simulink model "tenzo1_05"  (Simulink 7.9)
settings: Solver=ode45  StartTime=0.0  StopTime=20  RelTol=1e-3
values from neighbouring files (symbols this model uses):
  A = [0 0 0 0 0 0 0 -9.80999999984 0 0 0 0 ... (144 elements, 12x12)]    [A.mat]    (also in QuadLqrAstat105.m = loadA.A; Tenzo1_05.m = [ 0 0 0 1 0 0 0 0 0 0 0 0)
  Aoss = A-V*C    [QuadLqrAstat105.m]
  B = loadB.B    [QuadLqrAstat105.m]    (also in Tenzo1_05.m = [zeros(5,4))
  Boss = [B-V*D V]    [QuadLqrAstat105.m]
  Clocal = [ 0 0 0 0 0 0 1 0 0 0 0 0 ... (first row only)    [Tenzo1_05.m]
  Coss = eye(size(A))    [QuadLqrAstat105.m]
  D = [0 0 0 0 0 0 0 0 0 0 0 0 ... (48 elements, 12x4)]    [D.mat]    (also in QuadLqrAstat105.m = loadD.D; Tenzo1_05.m = zeros(4,4))
  Doss = zeros(size(Boss))    [QuadLqrAstat105.m]
  g = 9.81    [QuadLqrAstat105.m]    (also in Tenzo1_05.m; quadsys.m)
  If = -0.3559    [QuadLqrAstat105.m]    (also in Tenzo1_05.m)
  K = lqr(A,B,Q,R)    [QuadLqrAstat105.m]
  k1 = 1    [QuadLqrAstat105.m]    (also in Tenzo1_05.m)
  k2 = 1.8693    [QuadLqrAstat105.m]
  k3 = 2.0018    [QuadLqrAstat105.m]
  k4 = 1.9986    [QuadLqrAstat105.m]
  Kt = ct*rho*rp^4*pi()    [QuadLqrAstat105.m]
  Ktm = Km/Kt    [QuadLqrAstat105.m]
  lx = 28.8e-3    (= 0.0288)    [QuadLqrAstat105.m]    (also in Tenzo1_05.m)
  ly = 28.8e-3    (= 0.0288)    [QuadLqrAstat105.m]    (also in Tenzo1_05.m)
  mq = 0.82    [QuadLqrAstat105.m]    (also in Tenzo1_05.m = 1.2)
  pulseAmp = 100    [QuadLqrAstat105.m]
  PulseOff = 1    [QuadLqrAstat105.m]
  pulseP = 20    [QuadLqrAstat105.m]
  pulsePh = 7    [QuadLqrAstat105.m]
  PWM_max = 2200    [QuadLqrAstat105.m]
  tc = 0.436    [QuadLqrAstat105.m]
  w1 = 3050    [QuadLqrAstat105.m]
  w2 = 5820    [QuadLqrAstat105.m]
  w3 = 4250    [QuadLqrAstat105.m]
  w4 = 5940    [QuadLqrAstat105.m]
  X0c = 3950    [QuadLqrAstat105.m]
undefined symbols (not defined in the file or in its folder): magnitude, pulseP4, refs, sigbuilder_block
libraries: simulink x8, simulink_extras x8, vrlib x3, aerolibtransform2 x2, aerolib6dof2 x1
settings Model: Creator=userk  LastModifiedBy=userk
settings DataIOCC: ExternalInput=getinputstruct(op_trim5)  InitialState=getstatestruct(op_trim5)
settings CodeAppCC: CustomSymbolStrType=$N$R$M_T

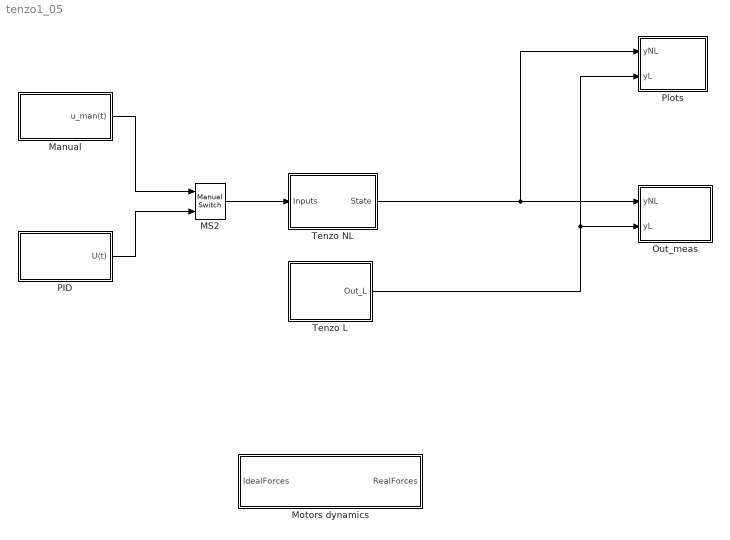
== system tenzo1_05 ==
  MS2 : simulink/Signal Routing/Manual Switch  sw=0  action=0  varsize=off
  Manual : Subsystem
  Motors dynamics : Subsystem
  Out_meas : Subsystem
  "PID " : Subsystem
  Plots : Subsystem
  Tenzo L : Subsystem
  Tenzo NL : Subsystem
  wires:
  Tenzo NL/1(State) -> Plots/1(yNL), Out_meas/1(yNL)
  MS2/1 -> Tenzo NL/1(Inputs)
  "PID "/1(U(t)) -> MS2/2
  Manual/1(u_man(t)) -> MS2/1
  Tenzo L/1(Out_L) -> Out_meas/2(yL), Plots/2(yL)

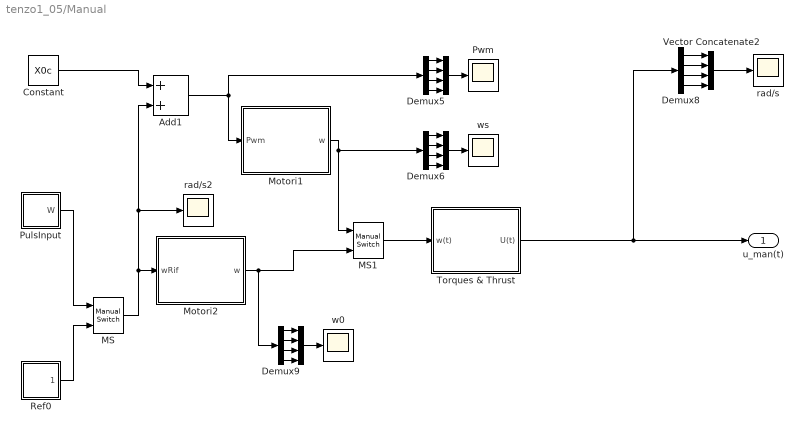
== system tenzo1_05/Manual ==
  " " : Concatenate  NumInputs=4
  "     " : Concatenate  NumInputs=4
  "                   " : Concatenate  NumInputs=4
  Add1 : Sum
  Constant : Constant  Value=X0c
  Demux{5..6,8..9} (4 alike) : Demux
  MS : simulink/Signal Routing/Manual Switch  sw=1  action=0  varsize=off
  MS1 : simulink/Signal Routing/Manual Switch  sw=0  action=0  varsize=off
  Motori1 : Subsystem
  Motori2 : Subsystem
  PulsInput : Subsystem
  Pwm : Scope
  Ref0 : Subsystem
  Torques & Thrust : Subsystem
  Vector Concatenate2 : Concatenate  NumInputs=4
  rad/s : Scope
      settings: YMin=0  YMax=8.5  SaveName=ScopeData12
  rad/s2 : Scope
      settings: YMin=3000  YMax=6000  SaveName=ScopeData3
  "w0  " : Scope
      settings: YMin=2500  YMax=7000  SaveName=ScopeData16
  ws : Scope
      settings: YMin=950  YMax=1950  SaveName=ScopeData10
  u_man(t) : Outport
  wires:
  Constant/1 -> Add1/1
  Add1/1 -> Motori1/1(Pwm), Demux5/1
  Motori1/1(w) -> Demux6/1, MS1/1
  Demux5/1 -> " "/1
  Demux5/2 -> " "/2
  Demux5/3 -> " "/3
  Demux5/4 -> " "/4
  " "/1 -> Pwm/1
  Demux6/1 -> "                   "/1
  Demux6/2 -> "                   "/2
  Demux6/3 -> "                   "/3
  Demux6/4 -> "                   "/4
  "                   "/1 -> ws/1
  MS1/1 -> Torques & Thrust/1(w(t))
  Demux8/1 -> Vector Concatenate2/1
  Demux8/2 -> Vector Concatenate2/2
  Demux8/3 -> Vector Concatenate2/3
  Demux8/4 -> Vector Concatenate2/4
  Vector Concatenate2/1 -> rad/s/1
  Motori2/1(w) -> Demux9/1, MS1/2
  Demux9/1 -> "     "/1
  Demux9/2 -> "     "/2
  Demux9/3 -> "     "/3
  Demux9/4 -> "     "/4
  "     "/1 -> "w0  "/1
  Torques & Thrust/1(U(t)) -> Demux8/1, u_man(t)/1
  Ref0/1(Out1) -> MS/2
  PulsInput/1(W) -> MS/1
  MS/1 -> Motori2/1(wRif), Add1/2, rad/s2/1

== system tenzo1_05/Motors dynamics ==
  IdealForces : Inport
  Demux11 : Demux
  Motors : Subsystem
  Mux3 : Mux
  T*toW : MATLAB Function  TreatAsAtomicUnit=on
  WtoTreal : Subsystem
  RealForces : Outport
  wires:
  Demux11/1 -> T*toW/1(T)
  Demux11/2 -> T*toW/2(taux)
  Demux11/3 -> T*toW/3(tauy)
  Demux11/4 -> T*toW/4(tauz)
  T*toW/1(w1) -> Mux3/1
  T*toW/2(w2) -> Mux3/2
  T*toW/3(w3) -> Mux3/3
  T*toW/4(w4) -> Mux3/4
  Mux3/1 -> Motors/1(wRif)
  Motors/1(w) -> WtoTreal/1(w(t))
  IdealForces/1 -> Demux11/1
  WtoTreal/1(U(t)) -> RealForces/1

== system tenzo1_05/Out_meas ==
  yNL : Inport
  yL : Inport  Port=2
  C : MATLAB Function  TreatAsAtomicUnit=on
  MS3 : simulink/Signal Routing/Manual Switch  sw=1  action=0  varsize=off
  To Workspace : ToWorkspace  VariableName=X  SampleTime=-1  SaveFormat=Timeseries
  "Ym(t) : output" : Scope
      settings: TimeRange=25  YMin=0  YMax=200  SaveName=ScopeData18
  Ymis : ToWorkspace  VariableName=Ymis  SampleTime=-1  SaveFormat=Timeseries
  wires:
  C/1(ymis) -> Ymis/1, "Ym(t) : output"/1
  MS3/1 -> C/1(X), To Workspace/1
  yNL/1 -> MS3/1
  yL/1 -> MS3/2

== system tenzo1_05/PID  ==
  Mux1 : Mux
  Pids : Subsystem
  Signal Builder : Subsystem  Tag=STV Subsys  LoadFcn=sigbuilder_block('load');  StartFcn=sigbuilder_block('start');  StopFcn=sigbuilder_block('stop');  ClipboardFcn=sigbuilder_block('clipboard');  mask(Sigbuilder block){}
      mask help: Simulink:masks:SigbuilderBlock_MD
      mask init:
      | if ~strcmp(get_param(bdroot(gcbh),'SimulationStatus'),'stopped') tuvar = sigbuilder_block('maskInit'); end
      settings: CopyFcn=sigbuilder_block('copy');  DeleteFcn=sigbuilder_block('delete');  ModelCloseFcn=sigbuilder_block('modelClose');  PreSaveFcn=sigbuilder_block('preSave');  PauseFcn=sigbuilder_block('pause');  ContinueFcn=sigbuilder_block('continue');  NameChangeFcn=sigbuilder_block('namechange');  OpenFcn=sigbuilder_block('open',[164 68 550.4 400 ]);  CloseFcn=sigbuilder_block('close');
      mask Display: plot(0, 0, 100, 100,[2, 2, 32, 32, 2], [68, 8, 8, 68, 68],[32, 2], [38, 38], [32, 19, 2],[53, 60, 44], [32, 17, 17, 2],[16, 16, 31, 31]);txt = getActiveGroup(gcbh);text(2, 100, txt,'verticalAlignment', 'top');
  Sum2 : Sum  Inputs=|++
  w0  2 : Scope
      settings: YMin=-2.75e+08  YMax=2.75e+08  SaveName=ScopeData35
  U(t) : Outport
  wires:
  Sum2/1 -> w0  2/1, U(t)/1
  Signal Builder/1(Thrust) -> Mux1/1
  Signal Builder/2(TauPhi) -> Mux1/2
  Signal Builder/3(TauTheta) -> Mux1/3
  Signal Builder/4(TauPsi) -> Mux1/4
  Mux1/1 -> Sum2/1
  Pids/1(u*(t)) -> Sum2/2

== system tenzo1_05/Plots ==
  yNL : Inport
  yL : Inport  Port=2
  Linear : Subsystem
  Non Linear : Subsystem
  VR Sink : vrlib/VR Sink  SampleTime=0.05  ViewEnable=on  RemoteChange=off  RemoteView=off  FieldsWritten=Lin.rotation.4.1.1.double#Lin.translation.3.1.1.double#NonLin.rotation.4.1.1.double#NonLin.translation.3.1.1.double  WorldFileName=aero.wrl  AutoView=off  VideoDimensions=[]  AllowVariableSize=off
  wires:
  yNL/1 -> Non Linear/1(y_nl)
  Linear/1(L rot) -> VR Sink/1
  yL/1 -> Linear/1(y_l)
  Non Linear/2(NL trasl) -> VR Sink/4
  Non Linear/1(NL rot) -> VR Sink/3
  Linear/2(L trasl) -> VR Sink/2

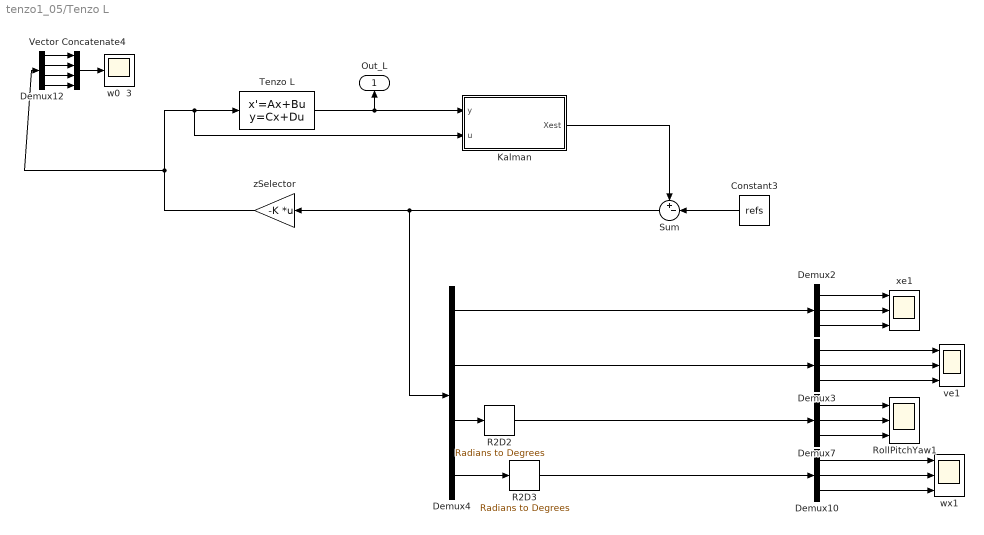
== system tenzo1_05/Tenzo L ==
  Constant3 : Constant  Value=refs
  Demux{2..3,7,10} (4 alike) : Demux  Outputs=3
  Demux12 : Demux
  Demux4 : Demux
  Kalman : Subsystem
  R2D2 : simulink_extras/Transformations/Radians to Degrees
  R2D3 : simulink_extras/Transformations/Radians to Degrees
  RollPitchYaw1 : Scope  NumInputPorts=3
      settings: YMin=-5~-5~-5  YMax=5~5~5  SaveName=ScopeData21
  Sum : Sum  Inputs=+-|
  Tenzo L : StateSpace  A=A  B=B  C=Clocal  D=D  X0=[0 0 -30 0 0 0 0 0 1 0 0 0]
  Vector Concatenate4 : Concatenate  NumInputs=4
  ve1 : Scope  NumInputPorts=3
      settings: YMin=-5~-5~-5  YMax=5~5~5  SaveName=ScopeData22
  w0  3 : Scope
      settings: YMin=2500  YMax=7000  SaveName=ScopeData36
  wx1 : Scope  NumInputPorts=3
      settings: TimeRange=15  YMin=-5~-5~-5  YMax=5~5~5  SaveName=ScopeData24
  xe1 : Scope  NumInputPorts=3
      settings: TimeRange=3  YMin=1.6e-05~1.6e-05~4.25e-17  YMax=3e-05~3e-05~7.75e-17  SaveName=ScopeData25
  zSelector : Gain  Gain=-K  Multiplication=Matrix(K*u)
  Out_L : Outport
  wires:
  Constant3/1 -> Sum/2
  Demux4/1 -> Demux2/1
  Demux4/2 -> Demux3/1
  Demux4/4 -> R2D3/1
  Demux2/1 -> xe1/1
  Demux2/2 -> xe1/2
  Demux2/3 -> xe1/3
  Demux3/1 -> ve1/1
  Demux3/2 -> ve1/2
  Demux3/3 -> ve1/3
  Demux7/1 -> RollPitchYaw1/1
  Demux10/1 -> wx1/1
  Demux7/2 -> RollPitchYaw1/2
  Demux7/3 -> RollPitchYaw1/3
  Demux10/2 -> wx1/2
  Demux10/3 -> wx1/3
  R2D2/1 -> Demux7/1
  R2D3/1 -> Demux10/1
  Demux4/3 -> R2D2/1
  Tenzo L/1 -> Kalman/1(y), Out_L/1
  zSelector/1 -> Demux12/1, Tenzo L/1, Kalman/2(u)
  Demux12/1 -> Vector Concatenate4/1
  Demux12/2 -> Vector Concatenate4/2
  Demux12/3 -> Vector Concatenate4/3
  Demux12/4 -> Vector Concatenate4/4
  Vector Concatenate4/1 -> w0  3/1
  Sum/1 -> zSelector/1, Demux4/1
  Kalman/1(Xest) -> Sum/1

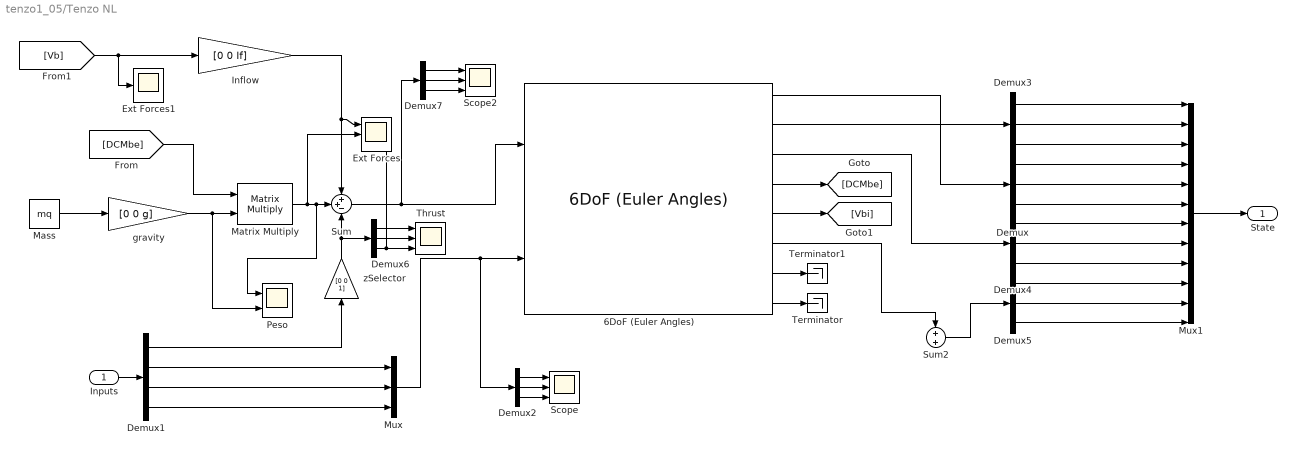
== system tenzo1_05/Tenzo NL ==
  Inputs : Inport
  6DoF (Euler Angles) : aerolib6dof2/6DoF (Euler Angles)  units=Metric (MKS)  mtype=Fixed  rep=Euler Angles  xme_0=[0 0 0]  Vm_0=[0 0 0]  eul_0=[0 0 0]  pm_0=[0 0 0]  mass_0=mq  mass_e=0.5  mass_f=2.0  inertia=II  inertia_e=eye(3)  inertia_f=2*eye(3)  k_quat=1.0
  Demux{,2..7} (7 alike) : Demux  Outputs=3
  Demux1 : Demux
  Ext Forces : Scope  NumInputPorts=3
      settings: TimeRange=30  YMin=-950000~-8~-5  YMax=0~2~5  SaveName=ScopeData5  SampleInput=on  SampleTime=0.01
  Ext Forces1 : Scope
      settings: TimeRange=30  YMin=-950000  YMax=0  SaveName=ScopeData27  SampleInput=on  SampleTime=0.01
  Inflow : Gain  Gain=[0 0 If]
  Mass : Constant  Value=mq
  Matrix Multiply : Product  Multiplication=Matrix(*)
  Mux : Mux  Inputs=3
  Mux1 : Mux  Inputs=12
  Peso : Scope  NumInputPorts=2
      settings: TimeRange=30  YMin=-8~0  YMax=2~8.5  SaveName=ScopeData8  SampleInput=on  SampleTime=0.01
  Scope : Scope  NumInputPorts=3
      settings: YMin=26050.4~-1~-671.375  YMax=28792.6~1~-607.435  SaveName=ScopeData4
  Scope2 : Scope  NumInputPorts=3
      settings: YMin=-1~-1~-2.3  YMax=1~1~-0.4  SaveName=ScopeData23
  Sum : Sum  Inputs=++-
  Sum2 : Sum
  Terminator : Terminator
  Terminator1 : Terminator
  Thrust : Scope  NumInputPorts=3
      settings: YMin=-1~-1~-2.3  YMax=1~1~-0.4  SaveName=ScopeData7
  gravity : Gain  Gain=[0 0 g]
  zSelector : Gain  Gain=[0 0 1]
  State : Outport
  wires:
  6DoF (Euler Angles)/4 -> [DCMbe]
  [DCMbe] -> Matrix Multiply/1
  Mass/1 -> gravity/1
  gravity/1 -> Matrix Multiply/2, Peso/2
  Matrix Multiply/1 -> Sum/2, Peso/1, Ext Forces/2
  6DoF (Euler Angles)/5 -> [Vbi]
  [Vb] -> Inflow/1, Ext Forces1/1
  Inflow/1 -> Sum/1, Ext Forces/1
  Demux1/1 -> zSelector/1
  Demux1/2 -> Mux/1
  Demux1/3 -> Mux/2
  Demux1/4 -> Mux/3
  Sum/1 -> Demux7/1, 6DoF (Euler Angles)/1
  Mux/1 -> 6DoF (Euler Angles)/2, Demux2/1
  6DoF (Euler Angles)/1 -> Demux/1
  6DoF (Euler Angles)/2 -> Demux3/1
  Demux3/1 -> Mux1/1
  Demux3/2 -> Mux1/2
  Demux3/3 -> Mux1/3
  Demux/1 -> Mux1/4
  Demux/2 -> Mux1/5
  Demux/3 -> Mux1/6
  Demux4/1 -> Mux1/7
  Demux4/2 -> Mux1/8
  Demux4/3 -> Mux1/9
  Demux5/1 -> Mux1/10
  Demux5/2 -> Mux1/11
  Demux5/3 -> Mux1/12
  6DoF (Euler Angles)/8 -> Terminator/1
  6DoF (Euler Angles)/7 -> Terminator1/1
  6DoF (Euler Angles)/3 -> Demux4/1
  Mux1/1 -> State/1
  Inputs/1 -> Demux1/1
  Demux2/1 -> Scope/1
  Demux2/2 -> Scope/2
  Demux2/3 -> Scope/3
  Demux7/1 -> Scope2/1
  Demux7/2 -> Scope2/2
  Demux7/3 -> Scope2/3
  zSelector/1 -> Sum/3, Demux6/1
  Demux6/1 -> Thrust/1
  Demux6/2 -> Thrust/2
  Demux6/3 -> Thrust/3, Ext Forces/3
  6DoF (Euler Angles)/6 -> Sum2/1
  Sum2/1 -> Demux5/1

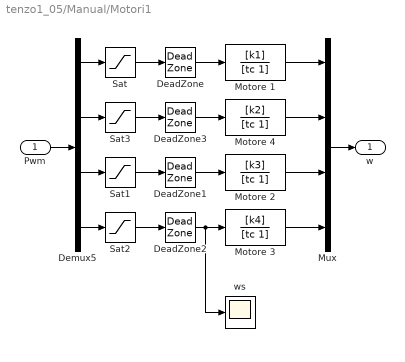
== system tenzo1_05/Manual/Motori1 ==
  Pwm : Inport
  DeadZone : DeadZone  LowerValue=0  UpperValue=dz1  SaturateOnIntegerOverflow=on
  DeadZone1 : DeadZone  LowerValue=0  UpperValue=dz3  SaturateOnIntegerOverflow=on
  DeadZone2 : DeadZone  LowerValue=0  UpperValue=dz4  SaturateOnIntegerOverflow=on
  DeadZone3 : DeadZone  LowerValue=0  UpperValue=dz2  SaturateOnIntegerOverflow=on
  Demux5 : Demux
  Motore 1 : TransferFcn  Numerator=[k1]  Denominator=[tc 1]
  Motore 2 : TransferFcn  Numerator=[k3]  Denominator=[tc 1]
  Motore 3 : TransferFcn  Numerator=[k4]  Denominator=[tc 1]
  Motore 4 : TransferFcn  Numerator=[k2]  Denominator=[tc 1]
  Mux : Mux
  Sat{,1..3} (4 alike) : Saturate  UpperLimit=PWM_max  LowerLimit=0
  ws : Scope
      settings: YMin=952.1  YMax=952.1  SaveName=ScopeData15
  w : Outport
  wires:
  Demux5/1 -> Sat/1
  Sat/1 -> DeadZone/1
  DeadZone/1 -> Motore 1/1
  Motore 1/1 -> Mux/1
  Sat1/1 -> DeadZone1/1
  DeadZone1/1 -> Motore 2/1
  Sat2/1 -> DeadZone2/1
  DeadZone2/1 -> Motore 3/1, ws/1
  Sat3/1 -> DeadZone3/1
  DeadZone3/1 -> Motore 4/1
  Demux5/2 -> Sat3/1
  Motore 4/1 -> Mux/2
  Demux5/3 -> Sat1/1
  Motore 2/1 -> Mux/3
  Demux5/4 -> Sat2/1
  Motore 3/1 -> Mux/4
  Pwm/1 -> Demux5/1
  Mux/1 -> w/1

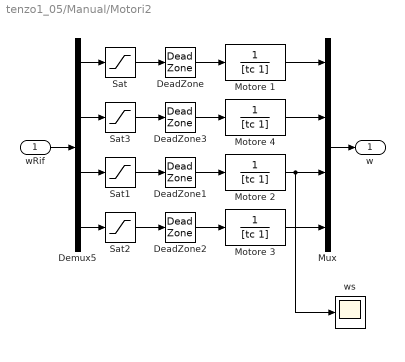
== system tenzo1_05/Manual/Motori2 ==
  wRif : Inport
  DeadZone{,1..3} (4 alike) : DeadZone  LowerValue=0  UpperValue=300  SaturateOnIntegerOverflow=on
  Demux5 : Demux
  Motore {1..4} (4 alike) : TransferFcn  Denominator=[tc 1]
  Mux : Mux
  Sat{,1..3} (4 alike) : Saturate  UpperLimit=10000  LowerLimit=0
  ws : Scope
      settings: YMin=904.495  YMax=999.705  SaveName=ScopeData15
  w : Outport
  wires:
  Mux/1 -> w/1
  wRif/1 -> Demux5/1
  Motore 3/1 -> Mux/4
  Demux5/4 -> Sat2/1
  Motore 2/1 -> Mux/3, ws/1
  Demux5/3 -> Sat1/1
  Motore 4/1 -> Mux/2
  Demux5/2 -> Sat3/1
  DeadZone3/1 -> Motore 4/1
  Sat3/1 -> DeadZone3/1
  DeadZone2/1 -> Motore 3/1
  Sat2/1 -> DeadZone2/1
  DeadZone1/1 -> Motore 2/1
  Sat1/1 -> DeadZone1/1
  Motore 1/1 -> Mux/1
  DeadZone/1 -> Motore 1/1
  Sat/1 -> DeadZone/1
  Demux5/1 -> Sat/1

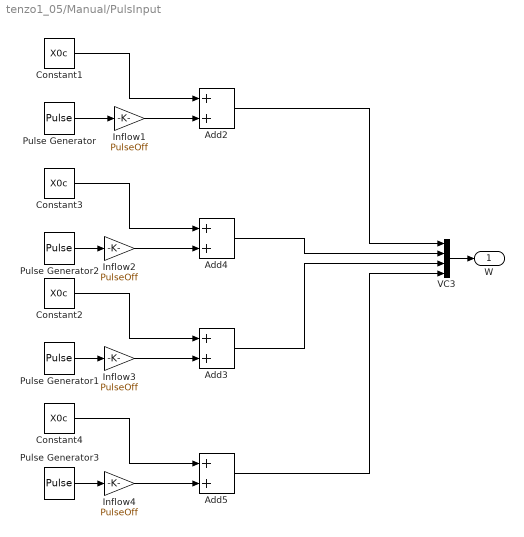
== system tenzo1_05/Manual/PulsInput ==
  Add{2..5} (4 alike) : Sum
  Constant{1..4} (4 alike) : Constant  Value=X0c
  Inflow{1..4} (4 alike) : Gain  Gain=PulseOff
  Pulse Generator : DiscretePulseGenerator  PulseType=Time based  Amplitude=pulseAmp  Period=pulseP  PulseWidth=50  PhaseDelay=pulsePh
  Pulse Generator1 : DiscretePulseGenerator  PulseType=Time based  Amplitude=pulseAmp  Period=pulseP  PulseWidth=50  PhaseDelay=pulsePh
  Pulse Generator2 : DiscretePulseGenerator  PulseType=Time based  Amplitude=pulseAmp  Period=pulseP  PulseWidth=50  PhaseDelay=pulsePh
  Pulse Generator3 : DiscretePulseGenerator  PulseType=Time based  Amplitude=pulseAmp  Period=pulseP4  PulseWidth=50  PhaseDelay=pulsePh
  VC3 : Concatenate  NumInputs=4
  W : Outport
  wires:
  Pulse Generator/1 -> Inflow1/1
  Constant1/1 -> Add2/1
  Pulse Generator1/1 -> Inflow3/1
  Constant2/1 -> Add3/1
  Pulse Generator2/1 -> Inflow2/1
  Constant3/1 -> Add4/1
  Pulse Generator3/1 -> Inflow4/1
  Constant4/1 -> Add5/1
  Add2/1 -> VC3/1
  Add4/1 -> VC3/2
  Add3/1 -> VC3/3
  Add5/1 -> VC3/4
  VC3/1 -> W/1
  Inflow1/1 -> Add2/2
  Inflow2/1 -> Add4/2
  Inflow3/1 -> Add3/2
  Inflow4/1 -> Add5/2

== system tenzo1_05/Manual/Ref0 ==
  Mux : Mux
  W1 : SignalGenerator  WaveForm=square  Amplitude=w1  Frequency=0.07
  W2 : SignalGenerator  WaveForm=square  Amplitude=w2  Frequency=0.07
  W3 : SignalGenerator  WaveForm=square  Amplitude=w3  Frequency=0.07
  W4 : SignalGenerator  WaveForm=square  Amplitude=w4  Frequency=0.07
  Out1 : Outport
  wires:
  W1/1 -> Mux/1
  W2/1 -> Mux/2
  W3/1 -> Mux/3
  W4/1 -> Mux/4
  Mux/1 -> Out1/1

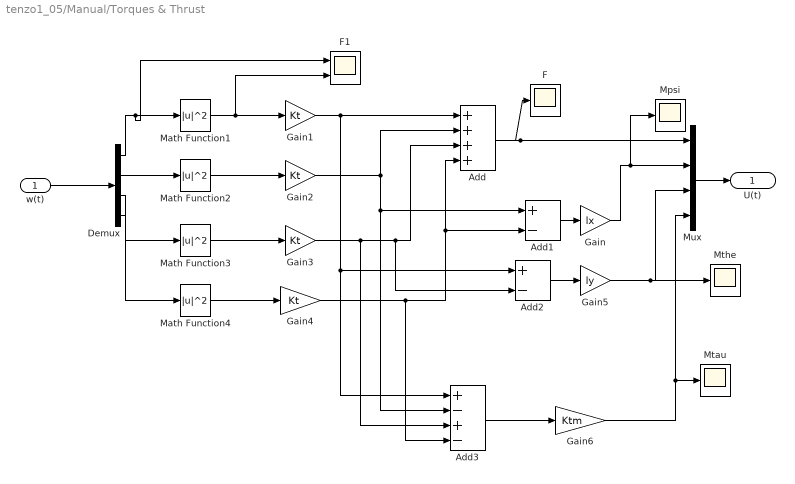
== system tenzo1_05/Manual/Torques & Thrust ==
  w(t) : Inport
  Add : Sum  Inputs=++++
  Add1 : Sum  Inputs=+-
  Add2 : Sum  Inputs=+-
  Add3 : Sum  Inputs=+-+-
  Demux : Demux
  F : Scope
      settings: SaveName=ScopeData17
  F1 : Scope  NumInputPorts=2
      settings: YMin=-5~-5  YMax=5~5  SaveName=ScopeData19
  Gain : Gain  Gain=lx
  Gain{1..4} (4 alike) : Gain  Gain=Kt
  Gain5 : Gain  Gain=ly
  Gain6 : Gain  Gain=Ktm
  Math Function{1..4} (4 alike) : Math  Operator=magnitude^2  SaturateOnIntegerOverflow=on
  Mpsi : Scope
      settings: SaveName=ScopeData14
  Mtau : Scope
      settings: SaveName=ScopeData11
  Mthe : Scope
      settings: SaveName=ScopeData13
  Mux : Mux
  U(t) : Outport
  wires:
  Math Function1/1 -> Gain1/1, F1/2
  Math Function2/1 -> Gain2/1
  Math Function3/1 -> Gain3/1
  Math Function4/1 -> Gain4/1
  Gain1/1 -> Add/1, Add2/1, Add3/1
  Gain2/1 -> Add/2, Add1/1, Add3/2
  Gain3/1 -> Add/3, Add2/2, Add3/3
  Gain4/1 -> Add/4, Add1/2, Add3/4
  Add/1 -> Mux/1, F/1
  Add1/1 -> Gain/1
  Add2/1 -> Gain5/1
  Gain/1 -> Mux/2, Mpsi/1
  Gain5/1 -> Mux/3, Mthe/1
  Add3/1 -> Gain6/1
  Gain6/1 -> Mux/4, Mtau/1
  Demux/1 -> Math Function1/1, F1/1
  Demux/2 -> Math Function2/1
  Mux/1 -> U(t)/1
  Demux/3 -> Math Function3/1
  Demux/4 -> Math Function4/1
  w(t)/1 -> Demux/1

== system tenzo1_05/Motors dynamics/Motors ==
  wRif : Inport
  DZ{,1..3} (4 alike) : DeadZone  LowerValue=0  UpperValue=300  SaturateOnIntegerOverflow=on
  Demux5 : Demux
  Motore {1..4} (4 alike) : TransferFcn  Denominator=[tc 1]
  Mux : Mux
  Sat{,1..3} (4 alike) : Saturate  UpperLimit=10000  LowerLimit=0
  ws : Scope
      settings: YMin=904.495  YMax=999.705  SaveName=ScopeData15
  w : Outport
  wires:
  Mux/1 -> w/1
  wRif/1 -> Demux5/1
  Motore 3/1 -> Mux/4
  Demux5/4 -> Sat2/1
  Motore 2/1 -> Mux/3
  Demux5/3 -> Sat1/1
  Motore 4/1 -> Mux/2
  Demux5/2 -> Sat3/1
  DZ1/1 -> Motore 4/1
  Sat3/1 -> DZ1/1
  DZ3/1 -> Motore 3/1
  Sat2/1 -> DZ3/1
  DZ2/1 -> Motore 2/1
  Sat1/1 -> DZ2/1
  Motore 1/1 -> Mux/1, ws/1
  DZ/1 -> Motore 1/1
  Sat/1 -> DZ/1
  Demux5/1 -> Sat/1

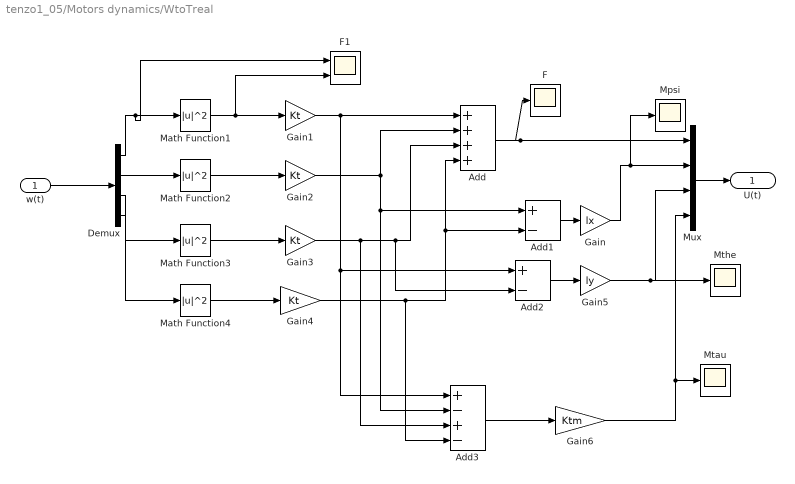
== system tenzo1_05/Motors dynamics/WtoTreal ==
  w(t) : Inport
  Add : Sum  Inputs=++++
  Add1 : Sum  Inputs=+-
  Add2 : Sum  Inputs=+-
  Add3 : Sum  Inputs=+-+-
  Demux : Demux
  F : Scope
      settings: SaveName=ScopeData17
  F1 : Scope  NumInputPorts=2
      settings: YMin=-5~-5  YMax=5~5  SaveName=ScopeData19
  Gain : Gain  Gain=lx
  Gain{1..4} (4 alike) : Gain  Gain=Kt
  Gain5 : Gain  Gain=ly
  Gain6 : Gain  Gain=Ktm
  Math Function{1..4} (4 alike) : Math  Operator=magnitude^2  SaturateOnIntegerOverflow=on
  Mpsi : Scope
      settings: SaveName=ScopeData14
  Mtau : Scope
      settings: SaveName=ScopeData11
  Mthe : Scope
      settings: SaveName=ScopeData13
  Mux : Mux
  U(t) : Outport
  wires:
  Math Function1/1 -> Gain1/1, F1/2
  Math Function2/1 -> Gain2/1
  Math Function3/1 -> Gain3/1
  Math Function4/1 -> Gain4/1
  Gain1/1 -> Add/1, Add2/1, Add3/1
  Gain2/1 -> Add/2, Add1/1, Add3/2
  Gain3/1 -> Add/3, Add2/2, Add3/3
  Gain4/1 -> Add/4, Add1/2, Add3/4
  Add/1 -> Mux/1, F/1
  Add1/1 -> Gain/1
  Add2/1 -> Gain5/1
  Gain/1 -> Mux/2, Mpsi/1
  Gain5/1 -> Mux/3, Mthe/1
  Add3/1 -> Gain6/1
  Gain6/1 -> Mux/4, Mtau/1
  Demux/1 -> Math Function1/1, F1/1
  Demux/2 -> Math Function2/1
  Mux/1 -> U(t)/1
  Demux/3 -> Math Function3/1
  Demux/4 -> Math Function4/1
  w(t)/1 -> Demux/1

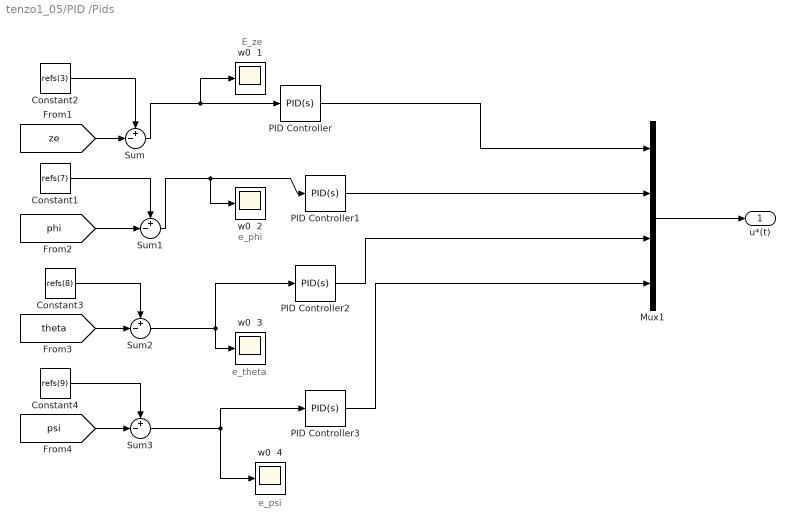
== system tenzo1_05/PID /Pids ==
  note: E_ze
  note: e_phi
  note: e_theta
  note: e_psi
  Constant1 : Constant  Value=refs(7)
  Constant2 : Constant  Value=refs(3)
  Constant3 : Constant  Value=refs(8)
  Constant4 : Constant  Value=refs(9)
  Mux1 : Mux
  PID Controller : simulink/Continuous/PID Controller  Controller=PID  TimeDomain=Continuous-time  SampleTime=1  IntegratorMethod=Forward Euler  FilterMethod=Forward Euler  Form=Parallel  P=-2.81657290050028  I=-0.10856097435728  D=-3.74671724354833  N=25.4035614147579  InitialConditionSource=internal  InitialConditionForIntegrator=0  InitialConditionForFilter=0  ExternalReset=none  LimitOutput=off  UpperSaturationLimit=inf  LowerSaturationLimit=-inf  LinearizeAsGain=off  AntiWindupMode=none  Kb=1  TrackingMode=off  Kt=1  PParamMin=[]  PParamMax=[]  IParamMin=[]  IParamMax=[]  DParamMin=[]  DParamMax=[]  NParamMin=[]  NParamMax=[]  KbParamMin=[]  KbParamMax=[]  KtParamMin=[]  KtParamMax=[]  POutMin=[]  POutMax=[]  IOutMin=[]  IOutMax=[]  DOutMin=[]  DOutMax=[]  NOutMin=[]  NOutMax=[]  KbOutMin=[]  KbOutMax=[]  KtOutMin=[]  KtOutMax=[]  IntegratorOutMin=[]  IntegratorOutMax=[]  FilterOutMin=[]  FilterOutMax=[]  SumOutMin=[]  SumOutMax=[]  SumI1OutMin=[]  SumI1OutMax=[]  SumI2OutMin=[]  SumI2OutMax=[]  SumI3OutMin=[]  SumI3OutMax=[]  SumDOutMin=[]  SumDOutMax=[]  SaturationOutMin=[]  SaturationOutMax=[]  IntegratorContinuousStateAttributes=''  IntegratorStateMustResolveToSignalObject=off  IntegratorRTWStateStorageClass=Auto  FilterContinuousStateAttributes=''  FilterStateMustResolveToSignalObject=off  FilterRTWStateStorageClass=Auto
  PID Controller1 : simulink/Continuous/PID Controller  Controller=PID  TimeDomain=Continuous-time  SampleTime=1  IntegratorMethod=Forward Euler  FilterMethod=Forward Euler  Form=Parallel  P=0.00227776084894012  I=0.000205170764798032  D=0.00233719169675889  N=31.074421221511  InitialConditionSource=internal  InitialConditionForIntegrator=0  InitialConditionForFilter=0  ExternalReset=none  LimitOutput=off  UpperSaturationLimit=inf  LowerSaturationLimit=-inf  LinearizeAsGain=off  AntiWindupMode=none  Kb=1  TrackingMode=off  Kt=1  PParamMin=[]  PParamMax=[]  IParamMin=[]  IParamMax=[]  DParamMin=[]  DParamMax=[]  NParamMin=[]  NParamMax=[]  KbParamMin=[]  KbParamMax=[]  KtParamMin=[]  KtParamMax=[]  POutMin=[]  POutMax=[]  IOutMin=[]  IOutMax=[]  DOutMin=[]  DOutMax=[]  NOutMin=[]  NOutMax=[]  KbOutMin=[]  KbOutMax=[]  KtOutMin=[]  KtOutMax=[]  IntegratorOutMin=[]  IntegratorOutMax=[]  FilterOutMin=[]  FilterOutMax=[]  SumOutMin=[]  SumOutMax=[]  SumI1OutMin=[]  SumI1OutMax=[]  SumI2OutMin=[]  SumI2OutMax=[]  SumI3OutMin=[]  SumI3OutMax=[]  SumDOutMin=[]  SumDOutMax=[]  SaturationOutMin=[]  SaturationOutMax=[]  IntegratorContinuousStateAttributes=''  IntegratorStateMustResolveToSignalObject=off  IntegratorRTWStateStorageClass=Auto  FilterContinuousStateAttributes=''  FilterStateMustResolveToSignalObject=off  FilterRTWStateStorageClass=Auto
  PID Controller2 : simulink/Continuous/PID Controller  Controller=PID  TimeDomain=Continuous-time  SampleTime=1  IntegratorMethod=Forward Euler  FilterMethod=Forward Euler  Form=Parallel  P=0.000563479429623525  I=3.39916753327837e-05  D=0.00199688923629926  N=54.5397025421619  InitialConditionSource=internal  InitialConditionForIntegrator=0  InitialConditionForFilter=0  ExternalReset=none  LimitOutput=off  UpperSaturationLimit=inf  LowerSaturationLimit=-inf  LinearizeAsGain=off  AntiWindupMode=none  Kb=1  TrackingMode=off  Kt=1  PParamMin=[]  PParamMax=[]  IParamMin=[]  IParamMax=[]  DParamMin=[]  DParamMax=[]  NParamMin=[]  NParamMax=[]  KbParamMin=[]  KbParamMax=[]  KtParamMin=[]  KtParamMax=[]  POutMin=[]  POutMax=[]  IOutMin=[]  IOutMax=[]  DOutMin=[]  DOutMax=[]  NOutMin=[]  NOutMax=[]  KbOutMin=[]  KbOutMax=[]  KtOutMin=[]  KtOutMax=[]  IntegratorOutMin=[]  IntegratorOutMax=[]  FilterOutMin=[]  FilterOutMax=[]  SumOutMin=[]  SumOutMax=[]  SumI1OutMin=[]  SumI1OutMax=[]  SumI2OutMin=[]  SumI2OutMax=[]  SumI3OutMin=[]  SumI3OutMax=[]  SumDOutMin=[]  SumDOutMax=[]  SaturationOutMin=[]  SaturationOutMax=[]  IntegratorContinuousStateAttributes=''  IntegratorStateMustResolveToSignalObject=off  IntegratorRTWStateStorageClass=Auto  FilterContinuousStateAttributes=''  FilterStateMustResolveToSignalObject=off  FilterRTWStateStorageClass=Auto
  PID Controller3 : simulink/Continuous/PID Controller  Controller=PID  TimeDomain=Continuous-time  SampleTime=1  IntegratorMethod=Forward Euler  FilterMethod=Forward Euler  Form=Parallel  P=0.000131344162662358  I=1.96774564028284e-06  D=0.000795936244237723  N=4.0451280111618  InitialConditionSource=internal  InitialConditionForIntegrator=0  InitialConditionForFilter=0  ExternalReset=none  LimitOutput=off  UpperSaturationLimit=inf  LowerSaturationLimit=-inf  LinearizeAsGain=off  AntiWindupMode=none  Kb=1  TrackingMode=off  Kt=1  PParamMin=[]  PParamMax=[]  IParamMin=[]  IParamMax=[]  DParamMin=[]  DParamMax=[]  NParamMin=[]  NParamMax=[]  KbParamMin=[]  KbParamMax=[]  KtParamMin=[]  KtParamMax=[]  POutMin=[]  POutMax=[]  IOutMin=[]  IOutMax=[]  DOutMin=[]  DOutMax=[]  NOutMin=[]  NOutMax=[]  KbOutMin=[]  KbOutMax=[]  KtOutMin=[]  KtOutMax=[]  IntegratorOutMin=[]  IntegratorOutMax=[]  FilterOutMin=[]  FilterOutMax=[]  SumOutMin=[]  SumOutMax=[]  SumI1OutMin=[]  SumI1OutMax=[]  SumI2OutMin=[]  SumI2OutMax=[]  SumI3OutMin=[]  SumI3OutMax=[]  SumDOutMin=[]  SumDOutMax=[]  SaturationOutMin=[]  SaturationOutMax=[]  IntegratorContinuousStateAttributes=''  IntegratorStateMustResolveToSignalObject=off  IntegratorRTWStateStorageClass=Auto  FilterContinuousStateAttributes=''  FilterStateMustResolveToSignalObject=off  FilterRTWStateStorageClass=Auto
  Sum{,1..3} (4 alike) : Sum  Inputs=+-|
  w0  {1..4} (4 alike) : Scope
      w0  1 settings: YMin=-2.5  YMax=-0.7  SaveName=ScopeData28
      w0  2 settings: YMin=2700  YMax=4700  SaveName=ScopeData32
      w0  3 settings: YMin=2700  YMax=4700  SaveName=ScopeData33
      w0  4 settings: YMin=2700  YMax=4700  SaveName=ScopeData34
  u*(t) : Outport
  wires:
  PID Controller3/1 -> Mux1/4
  Sum1/1 -> PID Controller1/1, w0  2/1
  Mux1/1 -> u*(t)/1
  Constant2/1 -> Sum/1
  [ze] -> Sum/2
  Sum/1 -> PID Controller/1, w0  1/1
  Constant1/1 -> Sum1/1
  [phi] -> Sum1/2
  Constant3/1 -> Sum2/1
  [theta] -> Sum2/2
  Sum2/1 -> PID Controller2/1, w0  3/1
  Constant4/1 -> Sum3/1
  [psi] -> Sum3/2
  Sum3/1 -> PID Controller3/1, w0  4/1
  PID Controller/1 -> Mux1/1
  PID Controller1/1 -> Mux1/2
  PID Controller2/1 -> Mux1/3

== system tenzo1_05/PID /Signal Builder ==
  Demux : Demux  Tag=STV Demux
  FromWs : FromWorkspace  Tag=STV FromWs  VariableName=tuvar  SampleTime=0  SigBuilderData=DataTag0  VnvData=DataTag1
      SigBuilderData=|
      | common.afterFinalStr = 'Extrapolate'
      | common.sampleTime = 0
      | dataSet.timeRange = [0 10]
      | dataSet.name = 'Group 1'
      | sbobj.Groups.Name = 'Group 1'
      | sbobj.Groups.Signals(1).Name = 'Thrust'
      | sbobj.Groups.Signals(1).XData = [0 10]
      | sbobj.Groups.Signals(1).YData = [0 0]
      | sbobj.Groups.Signals(2).Name = 'TauPhi'
      | sbobj.Groups.Signals(2).XData = [0 4 4 4.38 4.38 10]
      | sbobj.Groups.Signals(2).YData = [0 0 -0.0102 -0.0102 0 0]
      | sbobj.Groups.Signals(3).Name = 'TauTheta'
      | sbobj.Groups.Signals(3).XData = [0 8.56 8.56 9 9 10]
      | sbobj.Groups.Signals(3).YData = [0 0 0.0105 0.0105 0 0]
      | sbobj.Groups.Signals(4).Name = 'TauPsi'
      | sbobj.Groups.Signals(4).XData = [0 4 6 10]
      | sbobj.Groups.Signals(4).YData = [0 0 0 0]
  Thrust : Outport  Tag=STV Outport
  TauPhi : Outport  Tag=STV Outport  Port=2
  TauTheta : Outport  Tag=STV Outport  Port=3
  TauPsi : Outport  Tag=STV Outport  Port=4
  wires:
  FromWs/1 -> Demux/1
  Demux/1 -> Thrust/1
  Demux/2 -> TauPhi/1
  Demux/3 -> TauTheta/1
  Demux/4 -> TauPsi/1

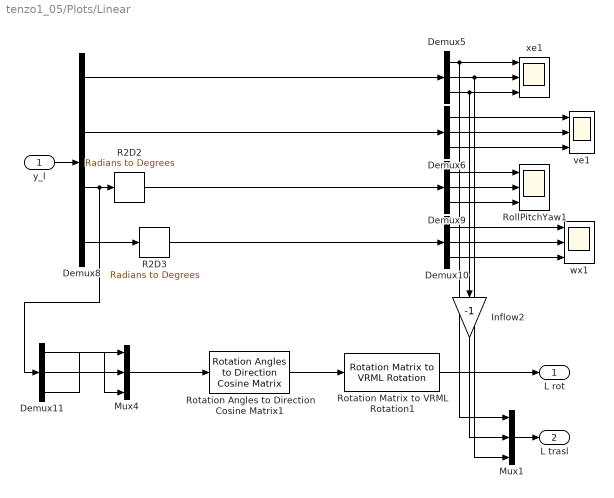
== system tenzo1_05/Plots/Linear ==
  y_l : Inport
  Demux{5..6,9..11} (5 alike) : Demux  Outputs=3
  Demux8 : Demux
  Inflow2 : Gain  Gain=-1
  Mux1 : Mux  Inputs=3
  Mux4 : Mux  Inputs=3
  R2D2 : simulink_extras/Transformations/Radians to Degrees
  R2D3 : simulink_extras/Transformations/Radians to Degrees
  RollPitchYaw1 : Scope  NumInputPorts=3
      settings: YMin=1000~1000~1000  YMax=2300~2300~2300  SaveName=ScopeData26
  Rotation Angles to Direction Cosine Matrix1 : aerolibtransform2/Rotation Angles to Direction Cosine Matrix  rotationOrder=ZYX
  Rotation Matrix to VRML Rotation1 : vrlib/Utilities/Rotation Matrix to VRML Rotation  maxzero=1e-12
  ve1 : Scope  NumInputPorts=3
      settings: YMin=-5~-5~-5  YMax=5~5~5  SaveName=ScopeData29
  wx1 : Scope  NumInputPorts=3
      settings: TimeRange=15  YMin=-5~-5~-5  YMax=5~5~5  SaveName=ScopeData30
  xe1 : Scope  NumInputPorts=3
      settings: TimeRange=15  YMin=4.25e-06~4.25e-06~-3.6e-14  YMax=7e-06~7e-06~-2.3e-14  SaveName=ScopeData31
  L rot : Outport
  L trasl : Outport  Port=2
  wires:
  Demux8/1 -> Demux5/1
  Demux8/2 -> Demux6/1
  Demux8/4 -> R2D3/1
  Demux5/1 -> Mux1/1, xe1/1
  Demux5/2 -> Mux1/3, xe1/2
  Demux5/3 -> xe1/3, Inflow2/1
  Demux6/1 -> ve1/1
  Demux6/2 -> ve1/2
  Demux6/3 -> ve1/3
  Demux9/1 -> RollPitchYaw1/1
  Demux10/1 -> wx1/1
  Demux9/2 -> RollPitchYaw1/2
  Demux9/3 -> RollPitchYaw1/3
  Demux10/2 -> wx1/2
  Demux10/3 -> wx1/3
  R2D2/1 -> Demux11/1, Demux9/1
  R2D3/1 -> Demux10/1
  Demux8/3 -> R2D2/1
  Rotation Angles to Direction Cosine Matrix1/1 -> Rotation Matrix to VRML Rotation1/1
  Mux4/1 -> Rotation Angles to Direction Cosine Matrix1/1
  Inflow2/1 -> Mux1/2
  Demux11/3 -> Mux4/1
  Demux11/2 -> Mux4/2
  Demux11/1 -> Mux4/3
  y_l/1 -> Demux8/1
  Rotation Matrix to VRML Rotation1/1 -> L rot/1
  Mux1/1 -> L trasl/1

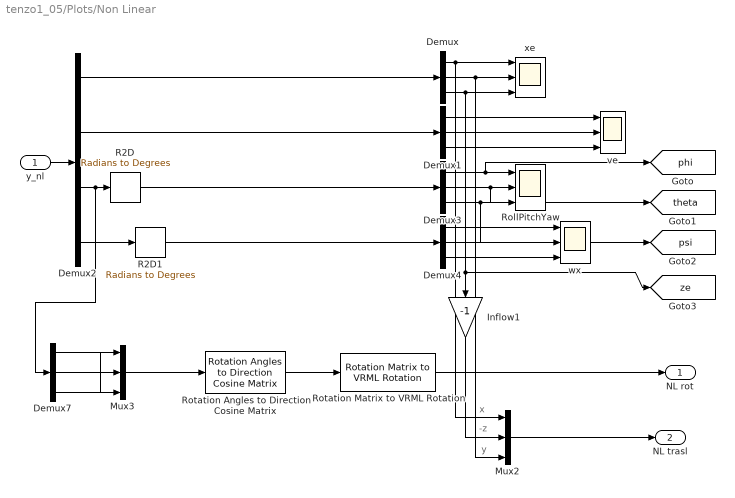
== system tenzo1_05/Plots/Non Linear ==
  note: -z
  note: x
  note: y
  y_nl : Inport
  Demux{,1,3..4,7} (5 alike) : Demux  Outputs=3
  Demux2 : Demux
  Inflow1 : Gain  Gain=-1
  Mux2 : Mux  Inputs=3
  Mux3 : Mux  Inputs=3
  R2D : simulink_extras/Transformations/Radians to Degrees
  R2D1 : simulink_extras/Transformations/Radians to Degrees
  RollPitchYaw : Scope  NumInputPorts=3
      settings: YMin=-1~-1~181.1  YMax=1~1~181.9  SaveName=ScopeData6
  Rotation Angles to Direction Cosine Matrix : aerolibtransform2/Rotation Angles to Direction Cosine Matrix  rotationOrder=ZYX
  Rotation Matrix to VRML Rotation : vrlib/Utilities/Rotation Matrix to VRML Rotation  maxzero=1e-12
  ve : Scope  NumInputPorts=3
      settings: YMin=-5~-5~-5  YMax=5~5~5  SaveName=ScopeData2
  wx : Scope  NumInputPorts=3
      settings: TimeRange=15  YMin=-2~-1.25~-0.07  YMax=2.5~3~0.02  SaveName=ScopeData9
  xe : Scope  NumInputPorts=3
      settings: TimeRange=3  YMin=-1~-1~-20  YMax=1~1~-12.5
  NL rot : Outport
  NL trasl : Outport  Port=2
  tag scope: phi=global, psi=global, theta=global, ze=global
  wires:
  Demux2/1 -> Demux/1
  Demux2/2 -> Demux1/1
  Demux2/4 -> R2D1/1
  Demux/1 -> xe/1, Mux2/1
  Demux/2 -> xe/2, Mux2/3
  Demux/3 -> xe/3, Inflow1/1, [ze]
  Demux1/1 -> ve/1
  Demux1/2 -> ve/2
  Demux1/3 -> ve/3
  Demux3/1 -> RollPitchYaw/1, [phi]
  Demux4/1 -> wx/1
  Demux3/2 -> RollPitchYaw/2, [theta]
  Demux3/3 -> RollPitchYaw/3, [psi]
  Demux4/2 -> wx/2
  Demux4/3 -> wx/3
  R2D/1 -> Demux3/1, Demux7/1
  R2D1/1 -> Demux4/1
  Demux2/3 -> R2D/1
  Rotation Angles to Direction Cosine Matrix/1 -> Rotation Matrix to VRML Rotation/1
  Mux3/1 -> Rotation Angles to Direction Cosine Matrix/1
  Inflow1/1 -> Mux2/2
  Demux7/2 -> Mux3/2
  Demux7/3 -> Mux3/1
  Demux7/1 -> Mux3/3
  y_nl/1 -> Demux2/1
  Rotation Matrix to VRML Rotation/1 -> NL rot/1
  Mux2/1 -> NL trasl/1

== system tenzo1_05/Tenzo L/Kalman ==
  note: 
  y : Inport
  u : Inport  Port=2
  Demux{,1,3..4} (4 alike) : Demux  Outputs=3
  Demux2 : Demux
  Kalman : Subsystem
  R2D : simulink_extras/Transformations/Radians to Degrees
  R2D1 : simulink_extras/Transformations/Radians to Degrees
  RollPitchYaw : Scope  NumInputPorts=3
      settings: YMin=-5~-5~-5  YMax=5~5~5  SaveName=ScopeData20
  Sum : Sum  Inputs=+-
  ve : Scope  NumInputPorts=3
      settings: YMin=-5~-5~-5  YMax=5~5~5  SaveName=ScopeData21
  wx : Scope  NumInputPorts=3
      settings: TimeRange=15  YMin=-5~-5~-5  YMax=5~5~5  SaveName=ScopeData22
  xe : Scope  NumInputPorts=3
      settings: TimeRange=15  YMin=-1e-14~-1.25e-14~-1e-18  YMax=1.25e-14~1.5e-14~8e-19  SaveName=ScopeData24
  Xest : Outport
  wires:
  Demux2/1 -> Demux/1
  Demux2/2 -> Demux1/1
  Demux2/4 -> R2D1/1
  Demux/1 -> xe/1
  Demux/2 -> xe/2
  Demux/3 -> xe/3
  Demux1/1 -> ve/1
  Demux1/2 -> ve/2
  Demux1/3 -> ve/3
  Demux3/1 -> RollPitchYaw/1
  Demux4/1 -> wx/1
  Demux3/2 -> RollPitchYaw/2
  Demux3/3 -> RollPitchYaw/3
  Demux4/2 -> wx/2
  Demux4/3 -> wx/3
  R2D/1 -> Demux3/1
  R2D1/1 -> Demux4/1
  Demux2/3 -> R2D/1
  Kalman/1(xi0) -> Xest/1, Sum/2
  Sum/1 -> Demux2/1
  u/1 -> Kalman/1(u)
  y/1 -> Kalman/2(y), Sum/1

== system tenzo1_05/Tenzo L/Kalman/Kalman ==
  u : Inport
  y : Inport  Port=2
  Mux : Mux  Inputs=[4 12]
  filtro di kalman : StateSpace  A=Aoss  B=Boss  C=Coss  D=Doss  X0=[0 0 0 0 0 0 0 0 0 0 0 0]
  xi0 : Outport
  wires:
  Mux/1 -> filtro di kalman/1
  u/1 -> Mux/1
  filtro di kalman/1 -> xi0/1
  y/1 -> Mux/2

== matlab function Motors dynamics/T*toW ==
  data: T input double; w1 output double; taux input double; tauy input double; tauz input double; w2 output double; w3 output double; w4 output double
function [w1,w2,w3,w4] = fcn(T,taux,tauy,tauz)
%#codegen
%% Physical properties of the environment
g=9.81; %Acceleration of gravity (m)
rho=1.2; %Density of air (m^3.kg^-1)

%% Physical properties of the quadrotor

% Total mass of the quadrotor [Kg]
mq=0.82;
% Motor length along x-axis (m). All motors have equal sizes.
lx=28.8e-3;
% Motor length along y-axis (m)
ly=28.8e-3;
% Motor length along z-axis (m)
lz=26e-3;

% Distance from the center of gravity to the center of a motor (m).
% The quadrotor is symmetric regarding the XZ and YZ planes, so
% dcg is the same for all motors.
dcg=0.288; 


% Inflow coefficient
If = -0.3559;

% Thrust coefficient of the propeller and Power coefficient
cp=0.0743; 
ct=0.1154;

% Propeller radius (m)
rp=25.4e-3; 
% Constant value to calculate the moment provided
% by a propeller given its angular speed (kg.m^2.rad^-1)
Km=cp*4*rho*rp^5/pi()^3; 
% Constant value to calculate the thrust provided
% by a propeller given its angular speed (kg.m.rad^-1) 
%Kt=ct*4*rho*rp^4/pi()^2; 
Kt=ct*rho*rp^4*pi();
% Constant that relates thrust and moment of a propeller.
Ktm=Km/Kt;
WTF = [ -Kt -Kt -Kt -Kt;
         0   -lx*Kt  0  lx*Kt;
        ly*Kt  0  -ly*Kt  0;
        Ktm -Ktm Ktm -Ktm];
    
    T= WTF^(-1)*[T; taux; tauy; tauz];
    w1 = T(1);
    w2 = T(2);
    w3 = T(3);
    w4 = T(4);

== matlab function Out_meas/C ==
  data: X input double; ymis output double
function ymis = fcn(X)
%#codegen

Cmis = [0 0 0 0 0 0 1 0 0 0 0 0;
        0 0 0 0 0 0 0 1 0 0 0 0;
        0 0 0 0 0 0 0 0 1 0 0 0;
        0 0 1 0 0 0 0 0 0 0 0 0];
ymis = Cmis*X;
